simulink model "half_adder"  (R2020b)
settings: Solver=VariableStepAuto  StartTime=0.0  StopTime=4  RelTol=1e-3
libraries: simulink x1, commutil2 x1
settings Model: Creator=hp  LastModifiedBy=hp

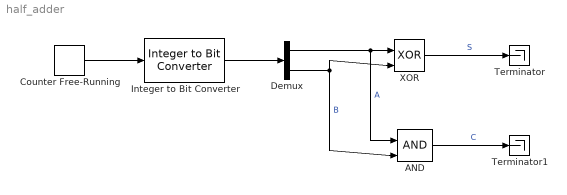
== system half_adder ==
  AND : Logic  IconShape=distinctive  AllPortsSameDT=off  OutDataTypeStr=boolean
  Counter Free-Running : simulink/Sources/Counter Free-Running  NumBits=2  tsamp=1
  Demux : Demux  Outputs=2
  Integer to Bit Converter : commutil2/Integer to Bit Converter  nbits=2  signedInputValues=Unsigned  bitOrder=MSB first  outDtype=Inherit via internal rule
  Terminator : Terminator
  Terminator1 : Terminator
  XOR : Logic  Operator=XOR  IconShape=distinctive  AllPortsSameDT=off  OutDataTypeStr=boolean
  wires:
  Counter Free-Running/1 -> Integer to Bit Converter/1
  Integer to Bit Converter/1 -> Demux/1
  Demux/1 -> AND/1, XOR/1  "A"
  Demux/2 -> AND/2, XOR/2  "B"
  XOR/1 -> Terminator/1  "S"
  AND/1 -> Terminator1/1  "C"
